simulink model "sm_vehicle_2axle_heave_roll_mu"  (R2024b)
settings: Solver=ode23t  StartTime=0.0  StopTime=14.2  MaxStep=0.2  RelTol=1e-3  AbsTol=1e-3  EnableMultiTasking=on
PostLoadFcn:
  | sm_vehicle_2axle_heave_roll_param
  | sm_vehicle_2axle_heave_roll_scene
  | sm_vehicle_2axle_heave_roll_config_maneuver(bdroot,VehicleData,'plateau');
  | set_param([bdroot '/Vehicle'],'popup_surface_conditions','Checker Right');
StartFcn:
  | tic
StopFcn:
  | Elapsed_Sim_Time = toc;
undefined symbols (not defined in the file): brake_trqTs, Disc, FL, FR, Hydraulic, InitVehicle, Mode, RL, RR, SceneData, valve_maxA, valve_maxO, VehicleData, X, Y, Z
libraries: fl_lib x92, sm_lib x43, nesl_utility x40, sm_vehicle_utilities_lib x21, sdl_lib x8, SimscapeFluids_lib x8, simulink x2, simulink_extras x1
(part 4 of 5)

== system sm_vehicle_2axle_heave_roll_mu/Brakes/Brake Control/Valve Open Loop/Mode to Valves RL ==
  note: Apply
  note: Hold
  note: Release
  C : Inport
  Constant : Constant  Value=[0 0]
  Constant1 : Constant  Value=[0 1]
  Constant2 : Constant  Value=[1 0]
  Multiport Switch : MultiPortSwitch  DataPortOrder=Zero-based contiguous  zeroidx=on  SaturateOnIntegerOverflow=off  InputSameDT=off
  V : Outport  VectorParamsAs1DForOutWhenUnconnected=off
  wires:
  Constant/1 -> Multiport Switch/2
  Constant1/1 -> Multiport Switch/3
  Constant2/1 -> Multiport Switch/4
  C/1 -> Multiport Switch/1
  Multiport Switch/1 -> V/1

== system sm_vehicle_2axle_heave_roll_mu/Brakes/Brake Control/Valve Open Loop/Mode to Valves RR ==
  note: Release
  note: Hold
  note: Apply
  C : Inport
  Constant : Constant  Value=[0 0]
  Constant1 : Constant  Value=[0 1]
  Constant2 : Constant  Value=[1 0]
  Multiport Switch : MultiPortSwitch  DataPortOrder=Zero-based contiguous  zeroidx=on  SaturateOnIntegerOverflow=off  InputSameDT=off
  V : Outport  VectorParamsAs1DForOutWhenUnconnected=off
  wires:
  Multiport Switch/1 -> V/1
  C/1 -> Multiport Switch/1
  Constant2/1 -> Multiport Switch/4
  Constant1/1 -> Multiport Switch/3
  Constant/1 -> Multiport Switch/2

== system sm_vehicle_2axle_heave_roll_mu/Brakes/Brakes/Damper/Actuator Dynamics FL ==
  In : Inport
  Gain : Gain  Gain=1./b
  Integrator : Integrator  InitialCondition=x_initial.*b
  Sum : Sum  Inputs=|+-  InputSameDT=on  SaturateOnIntegerOverflow=on  OutDataTypeStr=Inherit: Same as first input
  Out : Outport  VectorParamsAs1DForOutWhenUnconnected=off
  wires:
  Gain/1 -> Out/1, Sum/2
  Integrator/1 -> Gain/1
  In/1 -> Sum/1
  Sum/1 -> Integrator/1

== system sm_vehicle_2axle_heave_roll_mu/Brakes/Brakes/Damper/Actuator Dynamics FR ==
  In : Inport
  Gain : Gain  Gain=1./b
  Integrator : Integrator  InitialCondition=x_initial.*b
  Sum : Sum  Inputs=|+-  InputSameDT=on  SaturateOnIntegerOverflow=on  OutDataTypeStr=Inherit: Same as first input
  Out : Outport  VectorParamsAs1DForOutWhenUnconnected=off
  wires:
  Sum/1 -> Integrator/1
  In/1 -> Sum/1
  Integrator/1 -> Gain/1
  Gain/1 -> Sum/2, Out/1

== system sm_vehicle_2axle_heave_roll_mu/Brakes/Brakes/Damper/Actuator Dynamics RL ==
  In : Inport
  Gain : Gain  Gain=1./b
  Integrator : Integrator  InitialCondition=x_initial.*b
  Sum : Sum  Inputs=|+-  InputSameDT=on  SaturateOnIntegerOverflow=on  OutDataTypeStr=Inherit: Same as first input
  Out : Outport  VectorParamsAs1DForOutWhenUnconnected=off
  wires:
  Sum/1 -> Integrator/1
  In/1 -> Sum/1
  Integrator/1 -> Gain/1
  Gain/1 -> Sum/2, Out/1

== system sm_vehicle_2axle_heave_roll_mu/Brakes/Brakes/Damper/Actuator Dynamics RR ==
  In : Inport
  Gain : Gain  Gain=1./b
  Integrator : Integrator  InitialCondition=x_initial.*b
  Sum : Sum  Inputs=|+-  InputSameDT=on  SaturateOnIntegerOverflow=on  OutDataTypeStr=Inherit: Same as first input
  Out : Outport  VectorParamsAs1DForOutWhenUnconnected=off
  wires:
  Gain/1 -> Out/1, Sum/2
  Integrator/1 -> Gain/1
  In/1 -> Sum/1
  Sum/1 -> Integrator/1

== system sm_vehicle_2axle_heave_roll_mu/Brakes/Brakes/Damper/Sensing trq FL ==
  Ideal Torque Sensor : fl_lib/Mechanical/Mechanical Sensors/Ideal Torque Sensor
  PS-Simulink Converter : nesl_utility/PS-Simulink Converter  PhysicalDomain=network_engine_domain  SubClassName=ps_output  LeftPortType=input  RightPortType=output  PseudoPeriodic=off  Frequencies=[]  VectorFormat=1-D array  Unit=1  AffineConversion=off
  C : PMIOPort  Side=Right
  R : PMIOPort  Port=2  Side=Left
  trq : Outport  VectorParamsAs1DForOutWhenUnconnected=off
  wires:
  PS-Simulink Converter/1 -> trq/1  "trq"
  connections:
  Ideal Torque Sensor/RConn2 -- PS-Simulink Converter/LConn1
  Ideal Torque Sensor/LConn1 -- R/RConn1
  Ideal Torque Sensor/RConn1 -- C/RConn1

== system sm_vehicle_2axle_heave_roll_mu/Brakes/Brakes/Damper/Sensing trq FR ==
  Ideal Torque Sensor : fl_lib/Mechanical/Mechanical Sensors/Ideal Torque Sensor
  PS-Simulink Converter : nesl_utility/PS-Simulink Converter  PhysicalDomain=network_engine_domain  SubClassName=ps_output  LeftPortType=input  RightPortType=output  PseudoPeriodic=off  Frequencies=[]  VectorFormat=1-D array  Unit=1  AffineConversion=off
  C : PMIOPort  Side=Right
  R : PMIOPort  Port=2  Side=Left
  trq : Outport  VectorParamsAs1DForOutWhenUnconnected=off
  wires:
  PS-Simulink Converter/1 -> trq/1  "trq"
  connections:
  Ideal Torque Sensor/RConn1 -- C/RConn1
  Ideal Torque Sensor/LConn1 -- R/RConn1
  Ideal Torque Sensor/RConn2 -- PS-Simulink Converter/LConn1

== system sm_vehicle_2axle_heave_roll_mu/Brakes/Brakes/Damper/Sensing trq RL ==
  Ideal Torque Sensor : fl_lib/Mechanical/Mechanical Sensors/Ideal Torque Sensor
  PS-Simulink Converter : nesl_utility/PS-Simulink Converter  PhysicalDomain=network_engine_domain  SubClassName=ps_output  LeftPortType=input  RightPortType=output  PseudoPeriodic=off  Frequencies=[]  VectorFormat=1-D array  Unit=1  AffineConversion=off
  C : PMIOPort  Side=Right
  R : PMIOPort  Port=2  Side=Left
  trq : Outport  VectorParamsAs1DForOutWhenUnconnected=off
  wires:
  PS-Simulink Converter/1 -> trq/1  "trq"
  connections:
  Ideal Torque Sensor/RConn1 -- C/RConn1
  Ideal Torque Sensor/LConn1 -- R/RConn1
  Ideal Torque Sensor/RConn2 -- PS-Simulink Converter/LConn1

== system sm_vehicle_2axle_heave_roll_mu/Brakes/Brakes/Damper/Sensing trq RR ==
  Ideal Torque Sensor : fl_lib/Mechanical/Mechanical Sensors/Ideal Torque Sensor
  PS-Simulink Converter : nesl_utility/PS-Simulink Converter  PhysicalDomain=network_engine_domain  SubClassName=ps_output  LeftPortType=input  RightPortType=output  PseudoPeriodic=off  Frequencies=[]  VectorFormat=1-D array  Unit=1  AffineConversion=off
  C : PMIOPort  Side=Right
  R : PMIOPort  Port=2  Side=Left
  trq : Outport  VectorParamsAs1DForOutWhenUnconnected=off
  wires:
  PS-Simulink Converter/1 -> trq/1  "trq"
  connections:
  Ideal Torque Sensor/RConn2 -- PS-Simulink Converter/LConn1
  Ideal Torque Sensor/LConn1 -- R/RConn1
  Ideal Torque Sensor/RConn1 -- C/RConn1

== system sm_vehicle_2axle_heave_roll_mu/Brakes/Brakes/Disc/Actuator ==
  Valve : Inport
  BrkOn : Inport  Port=2
  Hydraulic : Subsystem  VariantControl=Hydraulic  mask(Ideal Hydraulic Caliper Actuators){brkTs=brake_trqTs, p_max=4e6, spr_rate=1e6, D=1e3}
      mask prompts: brkTs "Filter time constant"; p_max "Simulink:blkprm_prompts:GainGain"; spr_rate "Spring Rate (N/m)"; D "Damping coefficient"
      mask help: Braking system with ideal hydraulic caliper actuation. Assumes desired pressure is always available at the caliper, with a time constant for actuator dynamics. Used to size hydraulic components.
      mask TypeOptions brkTs:
      | Actuator
      | Dynamics FL/b | Actuator
      | Dynamics FR/b | Actuator
      | Dynamics RL/b | Actuator
      | Dynamics RR/b
      mask TypeOptions p_max: Gain FL/Gain | Gain FR/Gain | Gain RL/Gain | Gain RR/Gain
      mask TypeOptions spr_rate: Return Spring FL/Spring/spr_rate | Return Spring FR/Spring/spr_rate | Return Spring RL/Spring/spr_rate | Return Spring RR/Spring/spr_rate
      mask TypeOptions D: Return Spring FL/Damper/D | Return Spring FR/Damper/D | Return Spring RL/Damper/D | Return Spring RR/Damper/D
      mask DialogControl p_max Prompt: Gain:
      mask Display: image('sm_vehicle_2axle_brake_act_hydraulic.png')
  Ideal : Subsystem  VariantControl=Ideal  mask(Ideal Caliper Actuators){brkTs=brake_trqTs, p_max=4e6, d_caliper_bore_f=d_caliper_bore_f, d_caliper_bore_r=d_caliper_bore_r, spr_rate=1e6, D=1e3}
      mask prompts: brkTs "Filter time constant"; p_max "Simulink:blkprm_prompts:GainGain"; d_caliper_bore_f "Front Caliper Cylinder Bore (m)"; d_caliper_bore_r "Rear Caliper Cylinder Bore (m)"; spr_rate "Spring Rate (N/m)"; D "Damping coefficient"
      mask help: Braking system with ideal caliper actuators. Assumes desired force can always be applied at the caliper, with a time constant for actuator dynamics. Used to size caliper actuators.
      mask TypeOptions brkTs:
      | Actuator
      | Dynamics FL/b | Actuator
      | Dynamics FR/b | Actuator
      | Dynamics RL/b | Actuator
      | Dynamics RR/b
      mask TypeOptions p_max: Gain FL/Gain | Gain FR/Gain | Gain RL/Gain | Gain RR/Gain
      mask TypeOptions d_caliper_bore_f: Front Piston Area/Cylinder Bore/Value
      mask TypeOptions d_caliper_bore_r: Rear Piston Area/Cylinder Bore/Value
      mask TypeOptions spr_rate: Return Spring FL/Spring/spr_rate | Return Spring FR/Spring/spr_rate | Return Spring RL/Spring/spr_rate | Return Spring RR/Spring/spr_rate
      mask TypeOptions D: Return Spring FL/Damper/D | Return Spring FR/Damper/D | Return Spring RL/Damper/D | Return Spring RR/Damper/D
      mask DialogControl p_max Prompt: Gain:
      mask Display: image('sm_vehicle_2axle_brake_act_ideal.png')
  Valves : Subsystem  VariantControl=Valves  mask(Valve-Actuated Calipers){brkTs=brake_trqTs*0.1, p_max=4e6/3*3*3, spr_rate=1e6*2, D=1e2*10, area_max_apply=valve_maxA*1e-5, open_max_apply=valve_maxO, area_max_rel=valve_maxA*1e-5, open_max_rel=valve_maxO}
      mask prompts: brkTs "Filter time constant"; p_max "Simulink:blkprm_prompts:GainGain"; spr_rate "Spring Rate (N/m)"; D "Damping coefficient"; area_max_apply "Max Area Apply Valve (m^2)"; open_max_apply "Max Opening Apply Valve (m)"; area_max_rel "Max Area Release Valve (m^2)"; open_max_rel "Max Opening Release Valve (m)"
      mask help: Brake actuation system with valve-actuated piston calipers.
      mask TypeOptions brkTs:
      | Valves FL/Actuator
      | Dynamics/b | Valves FR/Actuator
      | Dynamics/b | Valves RL/Actuator
      | Dynamics/b | Valves RR/Actuator
      | Dynamics RR/b
      mask TypeOptions p_max: MC Pressure/Value
      mask TypeOptions spr_rate: Return Spring FL/Spring/spr_rate | Return Spring FR/Spring/spr_rate | Return Spring RL/Spring/spr_rate | Return Spring RR/Spring/spr_rate
      mask TypeOptions D: Return Spring FL/Damper/D | Return Spring FR/Damper/D | Return Spring RL/Damper/D | Return Spring RR/Damper/D
      mask DialogControl p_max Prompt: Gain:
      mask Display: image('sm_vehicle_2axle_brake_act_valves.png');
  pFL : PMIOPort  Side=Left
  pFR : PMIOPort  Port=2  Side=Right
  pRL : PMIOPort  Port=3  Side=Left
  pRR : PMIOPort  Port=4  Side=Right
  meas : Outport  VectorParamsAs1DForOutWhenUnconnected=off

== system sm_vehicle_2axle_heave_roll_mu/Brakes/Brakes/Disc/Sensing trq FL ==
  Ideal Torque Sensor : fl_lib/Mechanical/Mechanical Sensors/Ideal Torque Sensor
  PS-Simulink Converter : nesl_utility/PS-Simulink Converter  PhysicalDomain=network_engine_domain  SubClassName=ps_output  LeftPortType=input  RightPortType=output  PseudoPeriodic=off  Frequencies=[]  VectorFormat=1-D array  Unit=1  AffineConversion=off
  C : PMIOPort  Side=Right
  R : PMIOPort  Port=2  Side=Left
  trq : Outport  VectorParamsAs1DForOutWhenUnconnected=off
  wires:
  PS-Simulink Converter/1 -> trq/1  "trq"
  connections:
  Ideal Torque Sensor/RConn1 -- C/RConn1
  Ideal Torque Sensor/LConn1 -- R/RConn1
  Ideal Torque Sensor/RConn2 -- PS-Simulink Converter/LConn1

== system sm_vehicle_2axle_heave_roll_mu/Brakes/Brakes/Disc/Sensing trq FR ==
  Ideal Torque Sensor : fl_lib/Mechanical/Mechanical Sensors/Ideal Torque Sensor
  PS-Simulink Converter : nesl_utility/PS-Simulink Converter  PhysicalDomain=network_engine_domain  SubClassName=ps_output  LeftPortType=input  RightPortType=output  PseudoPeriodic=off  Frequencies=[]  VectorFormat=1-D array  Unit=1  AffineConversion=off
  C : PMIOPort  Side=Right
  R : PMIOPort  Port=2  Side=Left
  trq : Outport  VectorParamsAs1DForOutWhenUnconnected=off
  wires:
  PS-Simulink Converter/1 -> trq/1  "trq"
  connections:
  Ideal Torque Sensor/RConn2 -- PS-Simulink Converter/LConn1
  Ideal Torque Sensor/LConn1 -- R/RConn1
  Ideal Torque Sensor/RConn1 -- C/RConn1

== system sm_vehicle_2axle_heave_roll_mu/Brakes/Brakes/Disc/Sensing trq RL ==
  Ideal Torque Sensor : fl_lib/Mechanical/Mechanical Sensors/Ideal Torque Sensor
  PS-Simulink Converter : nesl_utility/PS-Simulink Converter  PhysicalDomain=network_engine_domain  SubClassName=ps_output  LeftPortType=input  RightPortType=output  PseudoPeriodic=off  Frequencies=[]  VectorFormat=1-D array  Unit=1  AffineConversion=off
  C : PMIOPort  Side=Right
  R : PMIOPort  Port=2  Side=Left
  trq : Outport  VectorParamsAs1DForOutWhenUnconnected=off
  wires:
  PS-Simulink Converter/1 -> trq/1  "trq"
  connections:
  Ideal Torque Sensor/RConn2 -- PS-Simulink Converter/LConn1
  Ideal Torque Sensor/LConn1 -- R/RConn1
  Ideal Torque Sensor/RConn1 -- C/RConn1

== system sm_vehicle_2axle_heave_roll_mu/Brakes/Brakes/Disc/Sensing trq RR ==
  Ideal Torque Sensor : fl_lib/Mechanical/Mechanical Sensors/Ideal Torque Sensor
  PS-Simulink Converter : nesl_utility/PS-Simulink Converter  PhysicalDomain=network_engine_domain  SubClassName=ps_output  LeftPortType=input  RightPortType=output  PseudoPeriodic=off  Frequencies=[]  VectorFormat=1-D array  Unit=1  AffineConversion=off
  C : PMIOPort  Side=Right
  R : PMIOPort  Port=2  Side=Left
  trq : Outport  VectorParamsAs1DForOutWhenUnconnected=off
  wires:
  PS-Simulink Converter/1 -> trq/1  "trq"
  connections:
  Ideal Torque Sensor/RConn1 -- C/RConn1
  Ideal Torque Sensor/LConn1 -- R/RConn1
  Ideal Torque Sensor/RConn2 -- PS-Simulink Converter/LConn1

== system sm_vehicle_2axle_heave_roll_mu/Brakes/Brake Control/Valve Closed Loop/Vehicle Speed/Dynamic Rate Limiter ==
  note: Y(k)
  note: U(k)
  up : Inport
  u : Inport  Port=2
  lo : Inport  Port=3
  Delay Input2 : UnitDelay  Description=Store in Global RAM  DisableCoverage=on  InitialCondition=InitVehicle.Vehicle.vx  SampleTime=-1  HasFrameUpgradeWarning=on
  Difference Inputs1 : Sum  Description=Add in CPU  DisableCoverage=on  Inputs=+-  OutDataTypeStr=Inherit: Inherit via back propagation
  Difference Inputs2 : Sum  Description=Add in CPU  OutDataTypeStr=Inherit: Inherit via back propagation
  FixPt Data Type Duplicate : DataTypeDuplicate  DisableCoverage=on  NumInputPorts=7
  Saturation Dynamic : simulink/Discontinuities/Saturation Dynamic  OutMin=[]  OutMax=[]  OutDataTypeStr=Inherit: Same as second input  OutDataType=fixdt(1, 16)  OutScaling=2^-10  DoSatur=off
  delta fall limit : Product  DisableCoverage=on  Inputs=**  OutDataTypeStr=Inherit: Inherit via back propagation  SaturateOnIntegerOverflow=on
  delta rise limit : Product  DisableCoverage=on  Inputs=**  OutDataTypeStr=Inherit: Inherit via back propagation  SaturateOnIntegerOverflow=on
  sample time : SampleTimeMath  DisableCoverage=on  TsampMathOp=Ts Only  weightValue=1
  Y : Outport  InitialOutput=0  VectorParamsAs1DForOutWhenUnconnected=off
  wires:
  Delay Input2/1 -> Difference Inputs1/2, FixPt Data Type Duplicate/2, Difference Inputs2/2  "Y(k-1)"
  sample time/1 -> delta fall limit/2, delta rise limit/2
  Difference Inputs2/1 -> Y/1, Delay Input2/1, FixPt Data Type Duplicate/1
  lo/1 -> delta fall limit/1
  up/1 -> delta rise limit/1
  delta rise limit/1 -> FixPt Data Type Duplicate/6, Saturation Dynamic/1
  Saturation Dynamic/1 -> Difference Inputs2/1, FixPt Data Type Duplicate/7
  Difference Inputs1/1 -> FixPt Data Type Duplicate/4, Saturation Dynamic/2  "( U(k) - Y(k-1) )"
  delta fall limit/1 -> FixPt Data Type Duplicate/3, Saturation Dynamic/3
  u/1 -> Difference Inputs1/1, FixPt Data Type Duplicate/5, sample time/1

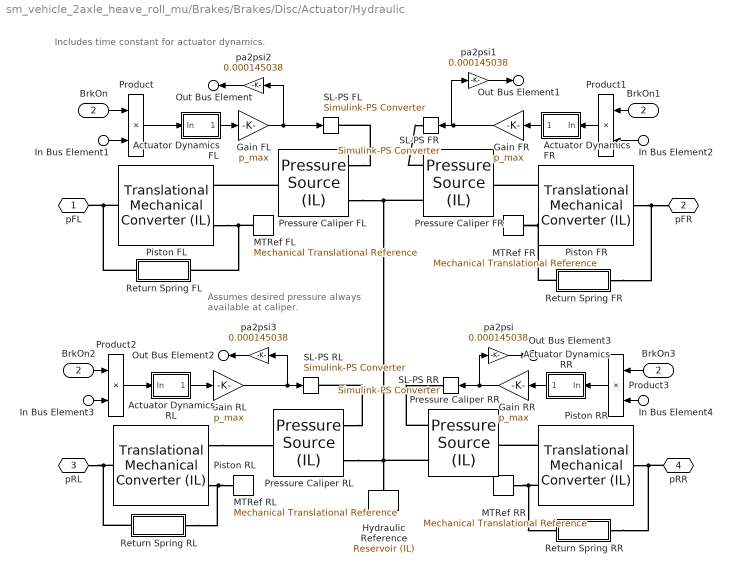
== system sm_vehicle_2axle_heave_roll_mu/Brakes/Brakes/Disc/Actuator/Hydraulic ==
  note: Includes time constant for actuator dynamics.
  note: Assumes desired pressure always available at caliper.
  In Bus Element1 : Inport  PortName=Valve  Element=FL
  In Bus Element2 : Inport  PortName=Valve  Element=FR
  In Bus Element3 : Inport  PortName=Valve  Element=RL
  In Bus Element4 : Inport  PortName=Valve  Element=RR
  BrkOn : Inport  Port=2
  Actuator Dynamics FL : Subsystem  mask(First-order lag supporting vector signals){b=brkTs, x_initial=0}
      mask prompts: b "Filter time constant"; x_initial "Initial output"
      mask help: Models a lag of the form 1/(b*s+1) where s is the Laplace operator.
  Actuator Dynamics FR : Subsystem  mask(First-order lag supporting vector signals){b=brkTs, x_initial=0}
      mask prompts: b "Filter time constant"; x_initial "Initial output"
      mask help: Models a lag of the form 1/(b*s+1) where s is the Laplace operator.
  Actuator Dynamics RL : Subsystem  mask(First-order lag supporting vector signals){b=brkTs, x_initial=0}
      mask prompts: b "Filter time constant"; x_initial "Initial output"
      mask help: Models a lag of the form 1/(b*s+1) where s is the Laplace operator.
  Actuator Dynamics RR : Subsystem  mask(First-order lag supporting vector signals){b=brkTs, x_initial=0}
      mask prompts: b "Filter time constant"; x_initial "Initial output"
      mask help: Models a lag of the form 1/(b*s+1) where s is the Laplace operator.
  BrkOn1 : InportShadow  Port=2
  BrkOn2 : InportShadow  Port=2
  BrkOn3 : InportShadow  Port=2
  Gain FL : Gain  Gain=p_max
  Gain FR : Gain  Gain=p_max
  Gain RL : Gain  Gain=p_max
  Gain RR : Gain  Gain=p_max
  Hydraulic Reference : fl_lib/Isothermal Liquid/Elements/Reservoir (IL)  reservoir_type=foundation.enum.constant_controlled.constant  pressure_spec=foundation.enum.pressure_spec.atmospheric  reservoir_pressure=0.101325 MPa
      settings: LibrarySourceBlock=fl_lib/Hydraulic/Hydraulic Elements/Hydraulic Reference
  MTRef FL : fl_lib/Mechanical/Translational Elements/Mechanical Translational Reference
  MTRef FR : fl_lib/Mechanical/Translational Elements/Mechanical Translational Reference
  MTRef RL : fl_lib/Mechanical/Translational Elements/Mechanical Translational Reference
  MTRef RR : fl_lib/Mechanical/Translational Elements/Mechanical Translational Reference
  Piston FL : fl_lib/Isothermal Liquid/Elements/Translational Mechanical Converter (IL)  mech_orientation=1  displacement_spec=foundation.enum.DisplacementSpec.Calculate  x0=0 m  interface_area=pist_area_pist_f m^2  dead_volume=1e-4 m^3  pressure_spec=1  environment_pressure=0.101325 MPa  dynamic_compressibility=1  p0=0 + 101325 Pa
      settings: InternalSimscapePortConfiguration="{\"Bottom\":[],\"Left\":[{\"id\":\"A\",\"label\":\"A\",\"type\":\"foundation.isothermal_liquid.isothermal_liquid\"},{\"id\":\"C\",\"label\":\"C\",\"type\":\"foundation.mechanical.translational.translational\"}],\"Right\":[{\"id\":\"R\",\"label\":\"R\",\"type\":\"foundation.mechanical.translational.translational\"}],\"Top\":[]}"
      settings: LibrarySourceBlock=|
      | fl_lib/Hydraulic/Hydraulic Elements/Translational
      | Hydro-Mechanical
      | Converter
  Piston FR : fl_lib/Isothermal Liquid/Elements/Translational Mechanical Converter (IL)  mech_orientation=1  displacement_spec=foundation.enum.DisplacementSpec.Calculate  x0=0 m  interface_area=pist_area_pist_f m^2  dead_volume=1e-4 m^3  pressure_spec=1  environment_pressure=0.101325 MPa  dynamic_compressibility=1  p0=0 + 101325 Pa
      settings: InternalSimscapePortConfiguration="{\"Bottom\":[],\"Left\":[{\"id\":\"A\",\"label\":\"A\",\"type\":\"foundation.isothermal_liquid.isothermal_liquid\"},{\"id\":\"C\",\"label\":\"C\",\"type\":\"foundation.mechanical.translational.translational\"}],\"Right\":[{\"id\":\"R\",\"label\":\"R\",\"type\":\"foundation.mechanical.translational.translational\"}],\"Top\":[]}"
      settings: LibrarySourceBlock=|
      | fl_lib/Hydraulic/Hydraulic Elements/Translational
      | Hydro-Mechanical
      | Converter
  Piston RL : fl_lib/Isothermal Liquid/Elements/Translational Mechanical Converter (IL)  mech_orientation=1  displacement_spec=foundation.enum.DisplacementSpec.Calculate  x0=0 m  interface_area=pist_area_pist_r m^2  dead_volume=1e-4 m^3  pressure_spec=1  environment_pressure=0.101325 MPa  dynamic_compressibility=1  p0=0 + 101325 Pa
      settings: InternalSimscapePortConfiguration="{\"Bottom\":[],\"Left\":[{\"id\":\"A\",\"label\":\"A\",\"type\":\"foundation.isothermal_liquid.isothermal_liquid\"},{\"id\":\"C\",\"label\":\"C\",\"type\":\"foundation.mechanical.translational.translational\"}],\"Right\":[{\"id\":\"R\",\"label\":\"R\",\"type\":\"foundation.mechanical.translational.translational\"}],\"Top\":[]}"
      settings: LibrarySourceBlock=|
      | fl_lib/Hydraulic/Hydraulic Elements/Translational
      | Hydro-Mechanical
      | Converter
  Piston RR : fl_lib/Isothermal Liquid/Elements/Translational Mechanical Converter (IL)  mech_orientation=1  displacement_spec=foundation.enum.DisplacementSpec.Calculate  x0=0 m  interface_area=pist_area_pist_r m^2  dead_volume=1e-4 m^3  pressure_spec=1  environment_pressure=0.101325 MPa  dynamic_compressibility=1  p0=0 + 101325 Pa
      settings: InternalSimscapePortConfiguration="{\"Bottom\":[],\"Left\":[{\"id\":\"A\",\"label\":\"A\",\"type\":\"foundation.isothermal_liquid.isothermal_liquid\"},{\"id\":\"C\",\"label\":\"C\",\"type\":\"foundation.mechanical.translational.translational\"}],\"Right\":[{\"id\":\"R\",\"label\":\"R\",\"type\":\"foundation.mechanical.translational.translational\"}],\"Top\":[]}"
      settings: LibrarySourceBlock=|
      | fl_lib/Hydraulic/Hydraulic Elements/Translational
      | Hydro-Mechanical
      | Converter
  Pressure Caliper FL : fl_lib/Isothermal Liquid/Sources/Pressure Source (IL)  source_type=foundation.enum.constant_controlled.controlled  pressure_differential=0 MPa
      settings: InternalSimscapePortConfiguration="{\"Bottom\":[],\"Left\":[{\"id\":\"A\",\"label\":\"A\",\"type\":\"foundation.isothermal_liquid.isothermal_liquid\"},{\"id\":\"P\",\"label\":\"P\",\"type\":\"input\"}],\"Right\":[{\"id\":\"B\",\"label\":\"B\",\"type\":\"foundation.isothermal_liquid.isothermal_liquid\"}],\"Top\":[]}"
      settings: LibrarySourceBlock=|
      | fl_lib/Hydraulic/Hydraulic Sources/Hydraulic Pressure
      | Source
  Pressure Caliper FR : fl_lib/Isothermal Liquid/Sources/Pressure Source (IL)  source_type=foundation.enum.constant_controlled.controlled  pressure_differential=0 MPa
      settings: InternalSimscapePortConfiguration="{\"Bottom\":[],\"Left\":[{\"id\":\"A\",\"label\":\"A\",\"type\":\"foundation.isothermal_liquid.isothermal_liquid\"},{\"id\":\"P\",\"label\":\"P\",\"type\":\"input\"}],\"Right\":[{\"id\":\"B\",\"label\":\"B\",\"type\":\"foundation.isothermal_liquid.isothermal_liquid\"}],\"Top\":[]}"
      settings: LibrarySourceBlock=|
      | fl_lib/Hydraulic/Hydraulic Sources/Hydraulic Pressure
      | Source
  Pressure Caliper RL : fl_lib/Isothermal Liquid/Sources/Pressure Source (IL)  source_type=foundation.enum.constant_controlled.controlled  pressure_differential=0 MPa
      settings: InternalSimscapePortConfiguration="{\"Bottom\":[],\"Left\":[{\"id\":\"A\",\"label\":\"A\",\"type\":\"foundation.isothermal_liquid.isothermal_liquid\"},{\"id\":\"P\",\"label\":\"P\",\"type\":\"input\"}],\"Right\":[{\"id\":\"B\",\"label\":\"B\",\"type\":\"foundation.isothermal_liquid.isothermal_liquid\"}],\"Top\":[]}"
      settings: LibrarySourceBlock=|
      | fl_lib/Hydraulic/Hydraulic Sources/Hydraulic Pressure
      | Source
  Pressure Caliper RR : fl_lib/Isothermal Liquid/Sources/Pressure Source (IL)  source_type=foundation.enum.constant_controlled.controlled  pressure_differential=0 MPa
      settings: InternalSimscapePortConfiguration="{\"Bottom\":[],\"Left\":[{\"id\":\"A\",\"label\":\"A\",\"type\":\"foundation.isothermal_liquid.isothermal_liquid\"},{\"id\":\"P\",\"label\":\"P\",\"type\":\"input\"}],\"Right\":[{\"id\":\"B\",\"label\":\"B\",\"type\":\"foundation.isothermal_liquid.isothermal_liquid\"}],\"Top\":[]}"
      settings: LibrarySourceBlock=|
      | fl_lib/Hydraulic/Hydraulic Sources/Hydraulic Pressure
      | Source
  Product{,1..3} (4 alike) : Product
  Return Spring FL : Subsystem
  Return Spring FR : Subsystem
  Return Spring RL : Subsystem
  Return Spring RR : Subsystem
  SL-PS FL : nesl_utility/Simulink-PS Converter  PhysicalDomain=network_engine_domain  SubClassName=ps_input  LeftPortType=input  RightPortType=output  PseudoPeriodic=off  Frequencies=[]  NoiseDistribution=none  NoiseParameters=[]  Unit=1  AffineConversion=off  FilteringAndDerivatives=filter  SimscapeFilterOrder=1  InputFilterTimeConstant=0.001  UdotUserProvided=0
  SL-PS FR : nesl_utility/Simulink-PS Converter  PhysicalDomain=network_engine_domain  SubClassName=ps_input  LeftPortType=input  RightPortType=output  PseudoPeriodic=off  Frequencies=[]  NoiseDistribution=none  NoiseParameters=[]  Unit=1  AffineConversion=off  FilteringAndDerivatives=filter  SimscapeFilterOrder=1  InputFilterTimeConstant=0.001  UdotUserProvided=0
  SL-PS RL : nesl_utility/Simulink-PS Converter  PhysicalDomain=network_engine_domain  SubClassName=ps_input  LeftPortType=input  RightPortType=output  PseudoPeriodic=off  Frequencies=[]  NoiseDistribution=none  NoiseParameters=[]  Unit=1  AffineConversion=off  FilteringAndDerivatives=filter  SimscapeFilterOrder=1  InputFilterTimeConstant=0.001  UdotUserProvided=0
  SL-PS RR : nesl_utility/Simulink-PS Converter  PhysicalDomain=network_engine_domain  SubClassName=ps_input  LeftPortType=input  RightPortType=output  PseudoPeriodic=off  Frequencies=[]  NoiseDistribution=none  NoiseParameters=[]  Unit=1  AffineConversion=off  FilteringAndDerivatives=filter  SimscapeFilterOrder=1  InputFilterTimeConstant=0.001  UdotUserProvided=0
  pa2psi{,1..3} (4 alike) : Gain  Gain=0.000145038
  pFL : PMIOPort  Side=Left
  pFR : PMIOPort  Port=2  Side=Right
  pRL : PMIOPort  Port=3  Side=Left
  pRR : PMIOPort  Port=4  Side=Right
  Out Bus Element : Outport  VectorParamsAs1DForOutWhenUnconnected=off  PortName=meas  Element=pFL
  Out Bus Element1 : Outport  VectorParamsAs1DForOutWhenUnconnected=off  PortName=meas  Element=pFR
  Out Bus Element2 : Outport  VectorParamsAs1DForOutWhenUnconnected=off  PortName=meas  Element=pRL
  Out Bus Element3 : Outport  VectorParamsAs1DForOutWhenUnconnected=off  PortName=meas  Element=pRR
  wires:
  Gain RL/1 -> pa2psi3/1, SL-PS RL/1
  Gain RR/1 -> pa2psi/1, SL-PS RR/1
  Gain FR/1 -> pa2psi1/1, SL-PS FR/1
  Gain FL/1 -> SL-PS FL/1, pa2psi2/1
  Product2/1 -> Actuator Dynamics RL/1(In)
  Product1/1 -> Actuator Dynamics FR/1(In)
  Actuator Dynamics RR/1(Out) -> Gain RR/1
  Product3/1 -> Actuator Dynamics RR/1(In)
  Actuator Dynamics RL/1(Out) -> Gain RL/1
  Product/1 -> Actuator Dynamics FL/1(In)
  Actuator Dynamics FL/1(Out) -> Gain FL/1
  Actuator Dynamics FR/1(Out) -> Gain FR/1
  In Bus Element1/1 -> Product/2
  BrkOn/1 -> Product/1
  BrkOn1/1 -> Product1/1
  In Bus Element2/1 -> Product1/2
  BrkOn2/1 -> Product2/1
  In Bus Element3/1 -> Product2/2
  BrkOn3/1 -> Product3/1
  In Bus Element4/1 -> Product3/2
  pa2psi/1 -> Out Bus Element3/1
  pa2psi1/1 -> Out Bus Element1/1
  pa2psi2/1 -> Out Bus Element/1
  pa2psi3/1 -> Out Bus Element2/1
  connections:
  Return Spring FR/LConn1 -- MTRef FR/LConn1 -- Piston FR/LConn2
  MTRef FL/LConn1 -- Piston FL/LConn2 -- Return Spring FL/LConn1
  Return Spring RL/LConn1 -- Piston RL/LConn2 -- MTRef RL/LConn1
  pFL/RConn1 -- Return Spring FL/RConn1 -- Piston FL/RConn1
  Return Spring FR/RConn1 -- Piston FR/RConn1 -- pFR/RConn1
  Return Spring RL/RConn1 -- pRL/RConn1 -- Piston RL/RConn1
  MTRef RR/LConn1 -- Return Spring RR/LConn1 -- Piston RR/LConn2
  Return Spring RR/RConn1 -- pRR/RConn1 -- Piston RR/RConn1
  Pressure Caliper FL/LConn2 -- SL-PS FL/RConn1
  Pressure Caliper FL/RConn1 -- Piston FL/LConn1
  Pressure Caliper FR/LConn2 -- SL-PS FR/RConn1
  Piston FR/LConn1 -- Pressure Caliper FR/RConn1
  Pressure Caliper RL/LConn2 -- SL-PS RL/RConn1
  Piston RL/LConn1 -- Pressure Caliper RL/RConn1
  Pressure Caliper FL/LConn1 -- Pressure Caliper FR/LConn1 -- Pressure Caliper RR/LConn1 -- Pressure Caliper RL/LConn1 -- Hydraulic Reference/LConn1
  Pressure Caliper RR/LConn2 -- SL-PS RR/RConn1
  Piston RR/LConn1 -- Pressure Caliper RR/RConn1

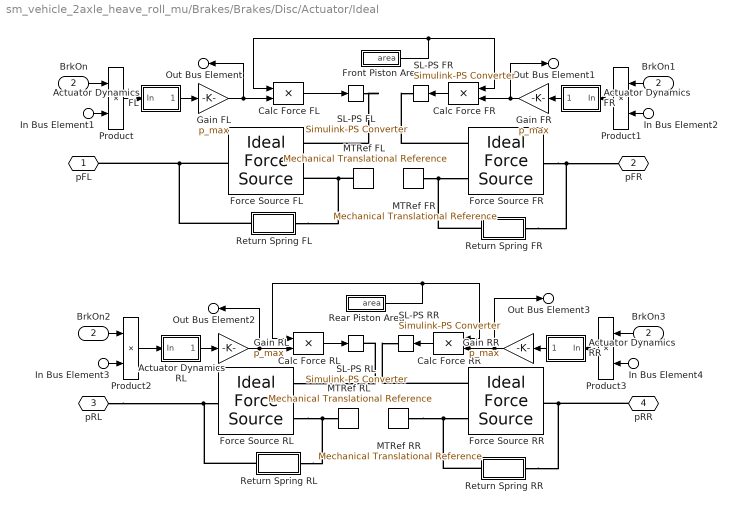
== system sm_vehicle_2axle_heave_roll_mu/Brakes/Brakes/Disc/Actuator/Ideal ==
  In Bus Element1 : Inport  PortName=Valve  Element=FL
  In Bus Element2 : Inport  PortName=Valve  Element=FR
  In Bus Element3 : Inport  PortName=Valve  Element=RL
  In Bus Element4 : Inport  PortName=Valve  Element=RR
  BrkOn : Inport  Port=2
  Actuator Dynamics FL : Subsystem  mask(First-order lag supporting vector signals){b=brkTs, x_initial=0}
      mask prompts: b "Filter time constant"; x_initial "Initial output"
      mask help: Models a lag of the form 1/(b*s+1) where s is the Laplace operator.
  Actuator Dynamics FR : Subsystem  mask(First-order lag supporting vector signals){b=brkTs, x_initial=0}
      mask prompts: b "Filter time constant"; x_initial "Initial output"
      mask help: Models a lag of the form 1/(b*s+1) where s is the Laplace operator.
  Actuator Dynamics RL : Subsystem  mask(First-order lag supporting vector signals){b=brkTs, x_initial=0}
      mask prompts: b "Filter time constant"; x_initial "Initial output"
      mask help: Models a lag of the form 1/(b*s+1) where s is the Laplace operator.
  Actuator Dynamics RR : Subsystem  mask(First-order lag supporting vector signals){b=brkTs, x_initial=0}
      mask prompts: b "Filter time constant"; x_initial "Initial output"
      mask help: Models a lag of the form 1/(b*s+1) where s is the Laplace operator.
  BrkOn1 : InportShadow  Port=2
  BrkOn2 : InportShadow  Port=2
  BrkOn3 : InportShadow  Port=2
  Calc Force FL : Product  Inputs=**
  Calc Force FR : Product  Inputs=**
  Calc Force RL : Product  Inputs=**
  Calc Force RR : Product  Inputs=**
  Force Source FL : fl_lib/Mechanical/Mechanical Sources/Ideal Force Source
  Force Source FR : fl_lib/Mechanical/Mechanical Sources/Ideal Force Source
  Force Source RL : fl_lib/Mechanical/Mechanical Sources/Ideal Force Source
  Force Source RR : fl_lib/Mechanical/Mechanical Sources/Ideal Force Source
  Front Piston Area : Subsystem
  Gain FL : Gain  Gain=p_max
  Gain FR : Gain  Gain=p_max
  Gain RL : Gain  Gain=p_max
  Gain RR : Gain  Gain=p_max
  MTRef FL : fl_lib/Mechanical/Translational Elements/Mechanical Translational Reference
  MTRef FR : fl_lib/Mechanical/Translational Elements/Mechanical Translational Reference
  MTRef RL : fl_lib/Mechanical/Translational Elements/Mechanical Translational Reference
  MTRef RR : fl_lib/Mechanical/Translational Elements/Mechanical Translational Reference
  Product{,1..3} (4 alike) : Product
  Rear Piston Area : Subsystem
  Return Spring FL : Subsystem
  Return Spring FR : Subsystem
  Return Spring RL : Subsystem
  Return Spring RR : Subsystem
  "SL-PS FL " : nesl_utility/Simulink-PS Converter  PhysicalDomain=network_engine_domain  SubClassName=ps_input  LeftPortType=input  RightPortType=output  PseudoPeriodic=off  Frequencies=[]  NoiseDistribution=none  NoiseParameters=[]  Unit=1  AffineConversion=off  FilteringAndDerivatives=filter  SimscapeFilterOrder=1  InputFilterTimeConstant=0.001  UdotUserProvided=0
  SL-PS FR : nesl_utility/Simulink-PS Converter  PhysicalDomain=network_engine_domain  SubClassName=ps_input  LeftPortType=input  RightPortType=output  PseudoPeriodic=off  Frequencies=[]  NoiseDistribution=none  NoiseParameters=[]  Unit=1  AffineConversion=off  FilteringAndDerivatives=filter  SimscapeFilterOrder=1  InputFilterTimeConstant=0.001  UdotUserProvided=0
  SL-PS RL : nesl_utility/Simulink-PS Converter  PhysicalDomain=network_engine_domain  SubClassName=ps_input  LeftPortType=input  RightPortType=output  PseudoPeriodic=off  Frequencies=[]  NoiseDistribution=none  NoiseParameters=[]  Unit=1  AffineConversion=off  FilteringAndDerivatives=filter  SimscapeFilterOrder=1  InputFilterTimeConstant=0.001  UdotUserProvided=0
  SL-PS RR : nesl_utility/Simulink-PS Converter  PhysicalDomain=network_engine_domain  SubClassName=ps_input  LeftPortType=input  RightPortType=output  PseudoPeriodic=off  Frequencies=[]  NoiseDistribution=none  NoiseParameters=[]  Unit=1  AffineConversion=off  FilteringAndDerivatives=filter  SimscapeFilterOrder=1  InputFilterTimeConstant=0.001  UdotUserProvided=0
  pFL : PMIOPort  Side=Left
  pFR : PMIOPort  Port=2  Side=Right
  pRL : PMIOPort  Port=3  Side=Left
  pRR : PMIOPort  Port=4  Side=Right
  Out Bus Element : Outport  VectorParamsAs1DForOutWhenUnconnected=off  PortName=meas  Element=pFL
  Out Bus Element1 : Outport  VectorParamsAs1DForOutWhenUnconnected=off  PortName=meas  Element=pFR
  Out Bus Element2 : Outport  VectorParamsAs1DForOutWhenUnconnected=off  PortName=meas  Element=pRL
  Out Bus Element3 : Outport  VectorParamsAs1DForOutWhenUnconnected=off  PortName=meas  Element=pRR
  wires:
  Actuator Dynamics FR/1(Out) -> Gain FR/1
  Actuator Dynamics FL/1(Out) -> Gain FL/1
  Product/1 -> Actuator Dynamics FL/1(In)
  Actuator Dynamics RL/1(Out) -> Gain RL/1
  Gain RL/1 -> Calc Force RL/2, Out Bus Element2/1
  Gain FL/1 -> Out Bus Element/1, Calc Force FL/2
  Product3/1 -> Actuator Dynamics RR/1(In)
  Actuator Dynamics RR/1(Out) -> Gain RR/1
  Gain RR/1 -> Out Bus Element3/1, Calc Force RR/2
  Gain FR/1 -> Calc Force FR/2, Out Bus Element1/1
  Product1/1 -> Actuator Dynamics FR/1(In)
  Product2/1 -> Actuator Dynamics RL/1(In)
  Calc Force FL/1 -> "SL-PS FL "/1
  Front Piston Area/1(area) -> Calc Force FL/1, Calc Force FR/1
  Calc Force FR/1 -> SL-PS FR/1
  Rear Piston Area/1(area) -> Calc Force RL/1, Calc Force RR/1
  Calc Force RR/1 -> SL-PS RR/1
  Calc Force RL/1 -> SL-PS RL/1
  BrkOn3/1 -> Product3/1
  BrkOn/1 -> Product/1
  BrkOn1/1 -> Product1/1
  BrkOn2/1 -> Product2/1
  In Bus Element1/1 -> Product/2
  In Bus Element3/1 -> Product2/2
  In Bus Element2/1 -> Product1/2
  In Bus Element4/1 -> Product3/2
  connections:
  "SL-PS FL "/RConn1 -- Force Source FL/RConn1
  Return Spring FL/LConn1 -- MTRef FL/LConn1 -- Force Source FL/RConn2
  Force Source FL/LConn1 -- Return Spring FL/RConn1 -- pFL/RConn1
  Force Source FR/LConn1 -- pFR/RConn1 -- Return Spring FR/RConn1
  Force Source FR/RConn1 -- SL-PS FR/RConn1
  Force Source RR/RConn1 -- SL-PS RR/RConn1
  Force Source RL/RConn1 -- SL-PS RL/RConn1
  pRR/RConn1 -- Return Spring RR/RConn1 -- Force Source RR/LConn1
  pRL/RConn1 -- Return Spring RL/RConn1 -- Force Source RL/LConn1
  Return Spring RL/LConn1 -- MTRef RL/LConn1 -- Force Source RL/RConn2
  Return Spring RR/LConn1 -- MTRef RR/LConn1 -- Force Source RR/RConn2
  Return Spring FR/LConn1 -- Force Source FR/RConn2 -- MTRef FR/LConn1

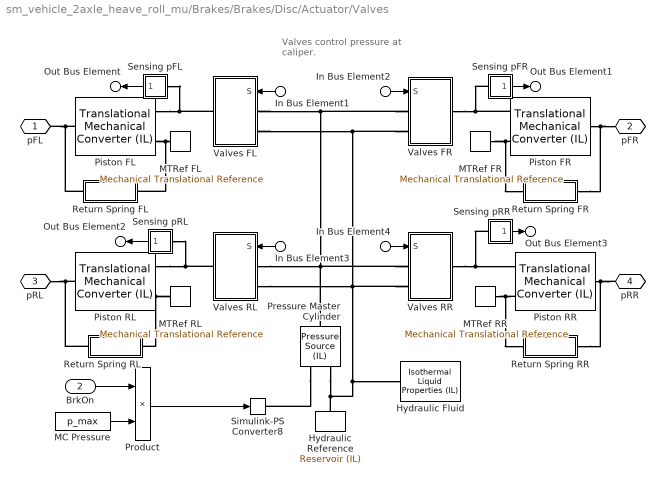
== system sm_vehicle_2axle_heave_roll_mu/Brakes/Brakes/Disc/Actuator/Valves ==
  note: Valves control pressure at caliper.
  In Bus Element1 : Inport  PortName=Valve  Element=FL
  In Bus Element2 : Inport  PortName=Valve  Element=FR
  In Bus Element3 : Inport  PortName=Valve  Element=RL
  In Bus Element4 : Inport  PortName=Valve  Element=RR
  BrkOn : Inport  Port=2
  Hydraulic Fluid : fl_lib/Isothermal Liquid/Utilities/Isothermal Liquid Properties (IL)  rho_L_atm=1001.952 kg/m^3  bulk_modulus_model=foundation.enum.bulk_modulus_model.const  beta_gain=6  beta_L_atm=1.52340e+09 Pa  nu_atm=(2.786)*(1) cSt  p_atm=0.101325 MPa  p_min=1 Pa  properties_range_check=simscape.enum.assert.action.error  air_fraction=0.005  polytropic_index=1.0  rho_g_atm=1.225 kg/m^3  air_dissolution_model=simscape.enum.onoff.off  p_crit=3 MPa
      settings: LibrarySourceBlock=sh_lib/Hydraulic Utilities/Hydraulic Fluid
  Hydraulic Reference : fl_lib/Isothermal Liquid/Elements/Reservoir (IL)  reservoir_type=foundation.enum.constant_controlled.constant  pressure_spec=foundation.enum.pressure_spec.atmospheric  reservoir_pressure=0.101325 MPa
      settings: LibrarySourceBlock=fl_lib/Hydraulic/Hydraulic Elements/Hydraulic Reference
  MC Pressure : Constant  Value=p_max
  MTRef FL : fl_lib/Mechanical/Translational Elements/Mechanical Translational Reference
  MTRef FR : fl_lib/Mechanical/Translational Elements/Mechanical Translational Reference
  MTRef RL : fl_lib/Mechanical/Translational Elements/Mechanical Translational Reference
  MTRef RR : fl_lib/Mechanical/Translational Elements/Mechanical Translational Reference
  Piston FL : fl_lib/Isothermal Liquid/Elements/Translational Mechanical Converter (IL)  mech_orientation=1  displacement_spec=foundation.enum.DisplacementSpec.Calculate  x0=0 m  interface_area=pist_area_pist_f m^2  dead_volume=1e-4 m^3  pressure_spec=1  environment_pressure=0.101325 MPa  dynamic_compressibility=1  p0=0 + 101325 Pa
      settings: InternalSimscapePortConfiguration="{\"Bottom\":[],\"Left\":[{\"id\":\"A\",\"label\":\"A\",\"type\":\"foundation.isothermal_liquid.isothermal_liquid\"},{\"id\":\"C\",\"label\":\"C\",\"type\":\"foundation.mechanical.translational.translational\"}],\"Right\":[{\"id\":\"R\",\"label\":\"R\",\"type\":\"foundation.mechanical.translational.translational\"}],\"Top\":[]}"
      settings: LibrarySourceBlock=|
      | fl_lib/Hydraulic/Hydraulic Elements/Translational
      | Hydro-Mechanical
      | Converter
  Piston FR : fl_lib/Isothermal Liquid/Elements/Translational Mechanical Converter (IL)  mech_orientation=1  displacement_spec=foundation.enum.DisplacementSpec.Calculate  x0=0 m  interface_area=pist_area_pist_f m^2  dead_volume=1e-4 m^3  pressure_spec=1  environment_pressure=0.101325 MPa  dynamic_compressibility=1  p0=0 + 101325 Pa
      settings: InternalSimscapePortConfiguration="{\"Bottom\":[],\"Left\":[{\"id\":\"A\",\"label\":\"A\",\"type\":\"foundation.isothermal_liquid.isothermal_liquid\"},{\"id\":\"C\",\"label\":\"C\",\"type\":\"foundation.mechanical.translational.translational\"}],\"Right\":[{\"id\":\"R\",\"label\":\"R\",\"type\":\"foundation.mechanical.translational.translational\"}],\"Top\":[]}"
      settings: LibrarySourceBlock=|
      | fl_lib/Hydraulic/Hydraulic Elements/Translational
      | Hydro-Mechanical
      | Converter
  Piston RL : fl_lib/Isothermal Liquid/Elements/Translational Mechanical Converter (IL)  mech_orientation=1  displacement_spec=foundation.enum.DisplacementSpec.Calculate  x0=0 m  interface_area=pist_area_pist_r m^2  dead_volume=1e-4 m^3  pressure_spec=1  environment_pressure=0.101325 MPa  dynamic_compressibility=1  p0=0 + 101325 Pa
      settings: InternalSimscapePortConfiguration="{\"Bottom\":[],\"Left\":[{\"id\":\"A\",\"label\":\"A\",\"type\":\"foundation.isothermal_liquid.isothermal_liquid\"},{\"id\":\"C\",\"label\":\"C\",\"type\":\"foundation.mechanical.translational.translational\"}],\"Right\":[{\"id\":\"R\",\"label\":\"R\",\"type\":\"foundation.mechanical.translational.translational\"}],\"Top\":[]}"
      settings: LibrarySourceBlock=|
      | fl_lib/Hydraulic/Hydraulic Elements/Translational
      | Hydro-Mechanical
      | Converter
  Piston RR : fl_lib/Isothermal Liquid/Elements/Translational Mechanical Converter (IL)  mech_orientation=1  displacement_spec=foundation.enum.DisplacementSpec.Calculate  x0=0 m  interface_area=pist_area_pist_r m^2  dead_volume=1e-4 m^3  pressure_spec=1  environment_pressure=0.101325 MPa  dynamic_compressibility=1  p0=0 + 101325 Pa
      settings: InternalSimscapePortConfiguration="{\"Bottom\":[],\"Left\":[{\"id\":\"A\",\"label\":\"A\",\"type\":\"foundation.isothermal_liquid.isothermal_liquid\"},{\"id\":\"C\",\"label\":\"C\",\"type\":\"foundation.mechanical.translational.translational\"}],\"Right\":[{\"id\":\"R\",\"label\":\"R\",\"type\":\"foundation.mechanical.translational.translational\"}],\"Top\":[]}"
      settings: LibrarySourceBlock=|
      | fl_lib/Hydraulic/Hydraulic Elements/Translational
      | Hydro-Mechanical
      | Converter
  Pressure Master Cylinder : fl_lib/Isothermal Liquid/Sources/Pressure Source (IL)  source_type=foundation.enum.constant_controlled.controlled  pressure_differential=0 MPa
      settings: InternalSimscapePortConfiguration="{\"Bottom\":[],\"Left\":[{\"id\":\"A\",\"label\":\"A\",\"type\":\"foundation.isothermal_liquid.isothermal_liquid\"},{\"id\":\"P\",\"label\":\"P\",\"type\":\"input\"}],\"Right\":[{\"id\":\"B\",\"label\":\"B\",\"type\":\"foundation.isothermal_liquid.isothermal_liquid\"}],\"Top\":[]}"
      settings: LibrarySourceBlock=|
      | fl_lib/Hydraulic/Hydraulic Sources/Hydraulic Pressure
      | Source
  Product : Product
  Return Spring FL : Subsystem
  Return Spring FR : Subsystem
  Return Spring RL : Subsystem
  Return Spring RR : Subsystem
  Sensing pFL : Subsystem
  Sensing pFR : Subsystem
  Sensing pRL : Subsystem
  Sensing pRR : Subsystem
  Simulink-PS Converter8 : nesl_utility/Simulink-PS Converter  PhysicalDomain=network_engine_domain  SubClassName=ps_input  LeftPortType=input  RightPortType=output  PseudoPeriodic=off  Frequencies=[]  NoiseDistribution=none  NoiseParameters=[]  Unit=1  AffineConversion=off  FilteringAndDerivatives=provide  SimscapeFilterOrder=1  InputFilterTimeConstant=0.001  UdotUserProvided=0
  Valves FL : Subsystem
  Valves FR : Subsystem
  Valves RL : Subsystem
  Valves RR : Subsystem
  pFL : PMIOPort  Side=Left
  pFR : PMIOPort  Port=2  Side=Right
  pRL : PMIOPort  Port=3  Side=Left
  pRR : PMIOPort  Port=4  Side=Right
  Out Bus Element : Outport  VectorParamsAs1DForOutWhenUnconnected=off  PortName=meas  Element=pFL
  Out Bus Element1 : Outport  VectorParamsAs1DForOutWhenUnconnected=off  PortName=meas  Element=pFR
  Out Bus Element2 : Outport  VectorParamsAs1DForOutWhenUnconnected=off  PortName=meas  Element=pRL
  Out Bus Element3 : Outport  VectorParamsAs1DForOutWhenUnconnected=off  PortName=meas  Element=pRR
  wires:
  Sensing pFL/1(p) -> Out Bus Element/1
  Sensing pFR/1(p) -> Out Bus Element1/1
  Sensing pRR/1(p) -> Out Bus Element3/1
  Sensing pRL/1(p) -> Out Bus Element2/1
  MC Pressure/1 -> Product/2
  In Bus Element1/1 -> Valves FL/1(S)
  In Bus Element2/1 -> Valves FR/1(S)
  In Bus Element4/1 -> Valves RR/1(S)
  In Bus Element3/1 -> Valves RL/1(S)
  BrkOn/1 -> Product/1
  Product/1 -> Simulink-PS Converter8/1
  connections:
  Valves RR/RConn1 -- Sensing pRR/LConn1 -- Piston RR/LConn1
  Valves RL/RConn1 -- Sensing pRL/LConn1 -- Piston RL/LConn1
  Piston FL/RConn1 -- Return Spring FL/RConn1 -- pFL/RConn1
  Return Spring FR/RConn1 -- Piston FR/RConn1 -- pFR/RConn1
  Valves FL/LConn1 -- Valves RL/LConn1 -- Pressure Master Cylinder/RConn1 -- Valves RR/LConn1 -- Valves FR/LConn1
  MTRef RL/LConn1 -- Piston RL/LConn2 -- Return Spring RL/LConn1
  MTRef FL/LConn1 -- Piston FL/LConn2 -- Return Spring FL/LConn1
  Sensing pFL/LConn1 -- Valves FL/RConn1 -- Piston FL/LConn1
  Valves FR/RConn1 -- Sensing pFR/LConn1 -- Piston FR/LConn1
  MTRef FR/LConn1 -- Piston FR/LConn2 -- Return Spring FR/LConn1
  Return Spring RL/RConn1 -- Piston RL/RConn1 -- pRL/RConn1
  MTRef RR/LConn1 -- Piston RR/LConn2 -- Return Spring RR/LConn1
  pRR/RConn1 -- Return Spring RR/RConn1 -- Piston RR/RConn1
  Valves FR/LConn2 -- Pressure Master Cylinder/LConn1 -- Hydraulic Reference/LConn1 -- Hydraulic Fluid/RConn1 -- Valves RL/LConn2 -- Valves RR/LConn2 -- Valves FL/LConn2
  Pressure Master Cylinder/LConn2 -- Simulink-PS Converter8/RConn1

== system sm_vehicle_2axle_heave_roll_mu/Brakes/Brakes/Disc/Actuator/Hydraulic/Actuator Dynamics FL ==
  In : Inport
  Gain : Gain  Gain=1./b
  Integrator : Integrator  InitialCondition=x_initial.*b
  Sum : Sum  Inputs=|+-  InputSameDT=on  SaturateOnIntegerOverflow=on  OutDataTypeStr=Inherit: Same as first input
  Out : Outport  VectorParamsAs1DForOutWhenUnconnected=off
  wires:
  Gain/1 -> Out/1, Sum/2
  Integrator/1 -> Gain/1
  In/1 -> Sum/1
  Sum/1 -> Integrator/1

== system sm_vehicle_2axle_heave_roll_mu/Brakes/Brakes/Disc/Actuator/Hydraulic/Actuator Dynamics FR ==
  In : Inport
  Gain : Gain  Gain=1./b
  Integrator : Integrator  InitialCondition=x_initial.*b
  Sum : Sum  Inputs=|+-  InputSameDT=on  SaturateOnIntegerOverflow=on  OutDataTypeStr=Inherit: Same as first input
  Out : Outport  VectorParamsAs1DForOutWhenUnconnected=off
  wires:
  Sum/1 -> Integrator/1
  In/1 -> Sum/1
  Integrator/1 -> Gain/1
  Gain/1 -> Sum/2, Out/1

== system sm_vehicle_2axle_heave_roll_mu/Brakes/Brakes/Disc/Actuator/Hydraulic/Actuator Dynamics RL ==
  In : Inport
  Gain : Gain  Gain=1./b
  Integrator : Integrator  InitialCondition=x_initial.*b
  Sum : Sum  Inputs=|+-  InputSameDT=on  SaturateOnIntegerOverflow=on  OutDataTypeStr=Inherit: Same as first input
  Out : Outport  VectorParamsAs1DForOutWhenUnconnected=off
  wires:
  Sum/1 -> Integrator/1
  In/1 -> Sum/1
  Integrator/1 -> Gain/1
  Gain/1 -> Sum/2, Out/1

== system sm_vehicle_2axle_heave_roll_mu/Brakes/Brakes/Disc/Actuator/Hydraulic/Actuator Dynamics RR ==
  In : Inport
  Gain : Gain  Gain=1./b
  Integrator : Integrator  InitialCondition=x_initial.*b
  Sum : Sum  Inputs=|+-  InputSameDT=on  SaturateOnIntegerOverflow=on  OutDataTypeStr=Inherit: Same as first input
  Out : Outport  VectorParamsAs1DForOutWhenUnconnected=off
  wires:
  Gain/1 -> Out/1, Sum/2
  Integrator/1 -> Gain/1
  In/1 -> Sum/1
  Sum/1 -> Integrator/1

== system sm_vehicle_2axle_heave_roll_mu/Brakes/Brakes/Disc/Actuator/Hydraulic/Return Spring FL ==
  Damper : fl_lib/Mechanical/Translational Elements/Translational Damper  D=D N/(m/s)  v_specify=off  v_priority=None  v=0 m/s  v_nominal_specify=off  v_nominal_value=1  v_nominal_unit=m/s  f_specify=off  f_priority=None  f=0 N  f_nominal_specify=off  f_nominal_value=1  f_nominal_unit=N
  Spring : fl_lib/Mechanical/Translational Elements/Translational Spring  spr_rate=spr_rate N/m  v_specify=off  v_priority=None  v=0 m/s  v_nominal_specify=off  v_nominal_value=1  v_nominal_unit=m/s  f_specify=off  f_priority=None  f=0 N  f_nominal_specify=off  f_nominal_value=1  f_nominal_unit=N  x_specify=off  x_priority=High  x=0 m  x_nominal_specify=off  x_nominal_value=1  x_nominal_unit=m
  R : PMIOPort  Side=Right
  C : PMIOPort  Port=2  Side=Left
  connections:
  Spring/RConn1 -- Damper/RConn1 -- C/RConn1
  Spring/LConn1 -- R/RConn1 -- Damper/LConn1

== system sm_vehicle_2axle_heave_roll_mu/Brakes/Brakes/Disc/Actuator/Hydraulic/Return Spring FR ==
  Damper : fl_lib/Mechanical/Translational Elements/Translational Damper  D=D N/(m/s)  v_specify=off  v_priority=None  v=0 m/s  v_nominal_specify=off  v_nominal_value=1  v_nominal_unit=m/s  f_specify=off  f_priority=None  f=0 N  f_nominal_specify=off  f_nominal_value=1  f_nominal_unit=N
  Spring : fl_lib/Mechanical/Translational Elements/Translational Spring  spr_rate=spr_rate N/m  v_specify=off  v_priority=None  v=0 m/s  v_nominal_specify=off  v_nominal_value=1  v_nominal_unit=m/s  f_specify=off  f_priority=None  f=0 N  f_nominal_specify=off  f_nominal_value=1  f_nominal_unit=N  x_specify=off  x_priority=High  x=0 m  x_nominal_specify=off  x_nominal_value=1  x_nominal_unit=m
  R : PMIOPort  Side=Right
  C : PMIOPort  Port=2  Side=Left
  connections:
  Damper/LConn1 -- R/RConn1 -- Spring/LConn1
  C/RConn1 -- Damper/RConn1 -- Spring/RConn1

== system sm_vehicle_2axle_heave_roll_mu/Brakes/Brakes/Disc/Actuator/Hydraulic/Return Spring RL ==
  Damper : fl_lib/Mechanical/Translational Elements/Translational Damper  D=D N/(m/s)  v_specify=off  v_priority=None  v=0 m/s  v_nominal_specify=off  v_nominal_value=1  v_nominal_unit=m/s  f_specify=off  f_priority=None  f=0 N  f_nominal_specify=off  f_nominal_value=1  f_nominal_unit=N
  Spring : fl_lib/Mechanical/Translational Elements/Translational Spring  spr_rate=spr_rate N/m  v_specify=off  v_priority=None  v=0 m/s  v_nominal_specify=off  v_nominal_value=1  v_nominal_unit=m/s  f_specify=off  f_priority=None  f=0 N  f_nominal_specify=off  f_nominal_value=1  f_nominal_unit=N  x_specify=off  x_priority=High  x=0 m  x_nominal_specify=off  x_nominal_value=1  x_nominal_unit=m
  R : PMIOPort  Side=Right
  C : PMIOPort  Port=2  Side=Left
  connections:
  R/RConn1 -- Damper/LConn1 -- Spring/LConn1
  C/RConn1 -- Spring/RConn1 -- Damper/RConn1

== system sm_vehicle_2axle_heave_roll_mu/Brakes/Brakes/Disc/Actuator/Hydraulic/Return Spring RR ==
  Damper : fl_lib/Mechanical/Translational Elements/Translational Damper  D=D N/(m/s)  v_specify=off  v_priority=None  v=0 m/s  v_nominal_specify=off  v_nominal_value=1  v_nominal_unit=m/s  f_specify=off  f_priority=None  f=0 N  f_nominal_specify=off  f_nominal_value=1  f_nominal_unit=N
  Spring : fl_lib/Mechanical/Translational Elements/Translational Spring  spr_rate=spr_rate N/m  v_specify=off  v_priority=None  v=0 m/s  v_nominal_specify=off  v_nominal_value=1  v_nominal_unit=m/s  f_specify=off  f_priority=None  f=0 N  f_nominal_specify=off  f_nominal_value=1  f_nominal_unit=N  x_specify=off  x_priority=High  x=0 m  x_nominal_specify=off  x_nominal_value=1  x_nominal_unit=m
  R : PMIOPort  Side=Right
  C : PMIOPort  Port=2  Side=Left
  connections:
  Spring/RConn1 -- Damper/RConn1 -- C/RConn1
  Spring/LConn1 -- R/RConn1 -- Damper/LConn1

== system sm_vehicle_2axle_heave_roll_mu/Brakes/Brakes/Disc/Actuator/Ideal/Actuator Dynamics FL ==
  In : Inport
  Gain : Gain  Gain=1./b
  Integrator : Integrator  InitialCondition=x_initial.*b
  Sum : Sum  Inputs=|+-  InputSameDT=on  SaturateOnIntegerOverflow=on  OutDataTypeStr=Inherit: Same as first input
  Out : Outport  VectorParamsAs1DForOutWhenUnconnected=off
  wires:
  Sum/1 -> Integrator/1
  In/1 -> Sum/1
  Integrator/1 -> Gain/1
  Gain/1 -> Sum/2, Out/1
